simulink model "Fieldcontrolmethod"  (Simulink 7.3)
settings: Solver=ode45  StartTime=0.0  StopTime=0.1  RelTol=1e-3
libraries: powerlib x7
settings Model: Creator=srija  LastModifiedBy=srija

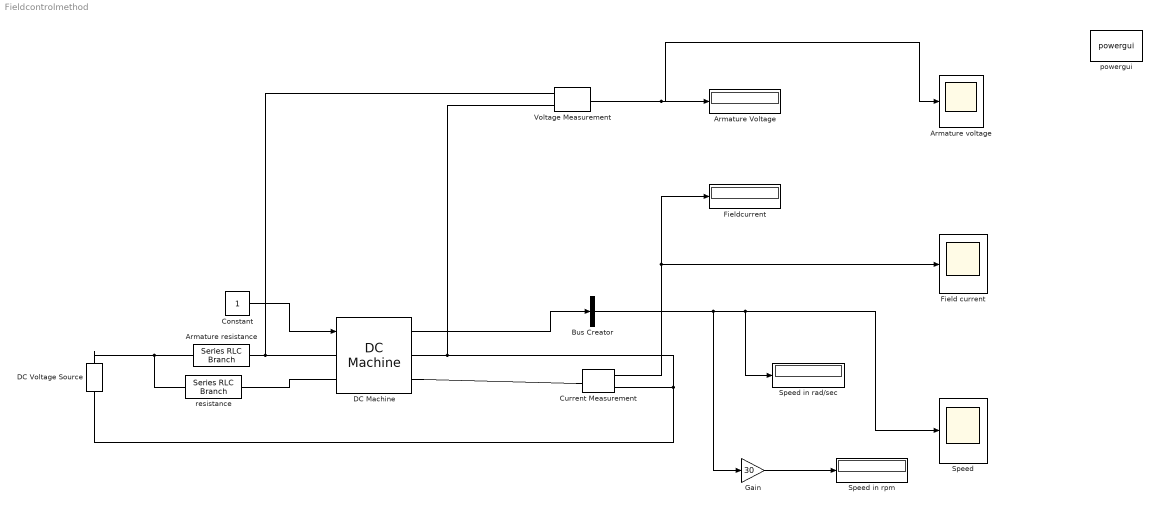
== system Fieldcontrolmethod ==
  Armature Voltage : Display
  Armature resistance : powerlib/Elements/Series RLC Branch  DialogController=POWERSYS.PowerSysDialog  PhysicalDomain=powersysdomain  SubClassName=unknown  LeftPortType=p1  RightPortType=p1  LConnTagsString=__new0  RConnTagsString=__new0  BranchType=R  Resistance=10  Inductance=1e-3  SetiL0=off  InitialCurrent=0  Capacitance=1e-6  Setx0=off  InitialVoltage=0  Measurements=None
  Armature voltage : Scope
  Bus Creator : BusCreator  Inputs=1
  Constant : Constant  OutDataType=fixdt(1, 16)  OutScaling=2^0
  Current Measurement : powerlib/Measurements/Current Measurement  DialogController=POWERSYS.PowerSysDialog  SystemSampleTime=-1  PhasorSimulation=off  OutputType=Complex  PSBequivalent=0
  DC Machine : powerlib/Machines/DC Machine  DialogController=POWERSYS.PowerSysDialog  SystemSampleTime=-1  PresetModel=No  MechanicalLoad=Torque TL  ShowDetailedParameters=on  RLa=[0.4832 0.006763]  RLf=[84.91 13.39]  Laf=0.7096  J=0.2053  Bm=0.007032  Tf=5.282  w0=0  Ifinit=2.8265221966476  TsPowergui=0  TsBlock=-1
  DC Voltage Source : powerlib/Electrical Sources/DC Voltage Source  DialogController=POWERSYS.PowerSysDialog  SystemSampleTime=-1  Amplitude=240  Measurements=None
  Field current : Scope
  "Fieldcurrent " : Display
  Gain : Gain  Gain=30  ParameterDataType=fixdt(1, 16)  ParameterScaling=2^0  OutDataType=fixdt(1, 16)  OutScaling=2^0
  Speed : Scope
      settings: SaveName=ScopeData2
  Speed in rad/sec : Display
  Speed in rpm : Display
  Voltage Measurement : powerlib/Measurements/Voltage Measurement  DialogController=POWERSYS.PowerSysDialog  SystemSampleTime=-1  PhasorSimulation=off  OutputType=Complex  PSBequivalent=0
  powergui : powerlib/powergui  Priority=1  SystemSampleTime=-1  SimulationMode=Continuous  SampleTime=50e-6  frequency=60  SPID=off  DisableSnubberDevices=off  DisableRonSwitches=off  DisableVfSwitches=off  SwTol=0  Interpol=off  frequencyindice=0  echomessages=off  HookPort=off  DisplayEquations=off  FunctionMessages=off  EnableUseOfTLC=off  x0status=blocks  RestoreLinks=warning  Frange=[0:2:500]  Ylog=off  Xlog=on  ShowGrid=off  save=off  variable=ZData  ZoomFFT=on  StartTime=0.0  cycles=1  DisplayStyle=1  fundamental=60  FreqAxis=off  MaxFrequency=1000  frequencyindicesteady=1  RmsSteady=1  display=off  Ts=0  methode=off
  resistance : powerlib/Elements/Series RLC Branch  DialogController=POWERSYS.PowerSysDialog  PhysicalDomain=powersysdomain  SubClassName=unknown  LeftPortType=p1  RightPortType=p1  LConnTagsString=__new0  RConnTagsString=__new0  BranchType=R  Resistance=0.0000001  Inductance=1e-3  SetiL0=off  InitialCurrent=0  Capacitance=1e-6  Setx0=off  InitialVoltage=0  Measurements=None
  wires:
  Voltage Measurement/1 -> Armature voltage/1, Armature Voltage/1
  Current Measurement/1 -> "Fieldcurrent "/1, Field current/1
  Constant/1 -> DC Machine/1
  DC Machine/1 -> Bus Creator/1
  Bus Creator/1 -> Speed/1, Speed in rad/sec/1, Gain/1
  Gain/1 -> Speed in rpm/1
  connections:
  DC Machine/RConn2 -- Current Measurement/LConn1
  DC Machine/RConn1 -- Current Measurement/RConn1 -- DC Voltage Source/LConn1 -- Voltage Measurement/LConn2
  Armature resistance/RConn1 -- DC Machine/LConn1 -- Voltage Measurement/LConn1
  resistance/RConn1 -- DC Machine/LConn2
  DC Voltage Source/RConn1 -- Armature resistance/LConn1 -- resistance/LConn1
